simulink model "test_dram_vacc_147"  (R2012b)
settings: Solver=VariableStepDiscrete  SolverMode=SingleTasking  StartTime=0.0  StopTime=100000  RelTol=1e-3
undefined symbols (not defined in the file): blockCountBits, blockRowBits
libraries: xbsIndex_r4 x1042, xbsReplacements_r4 x87, casper_library_misc x9, xps_library x2
(part 2 of 9)

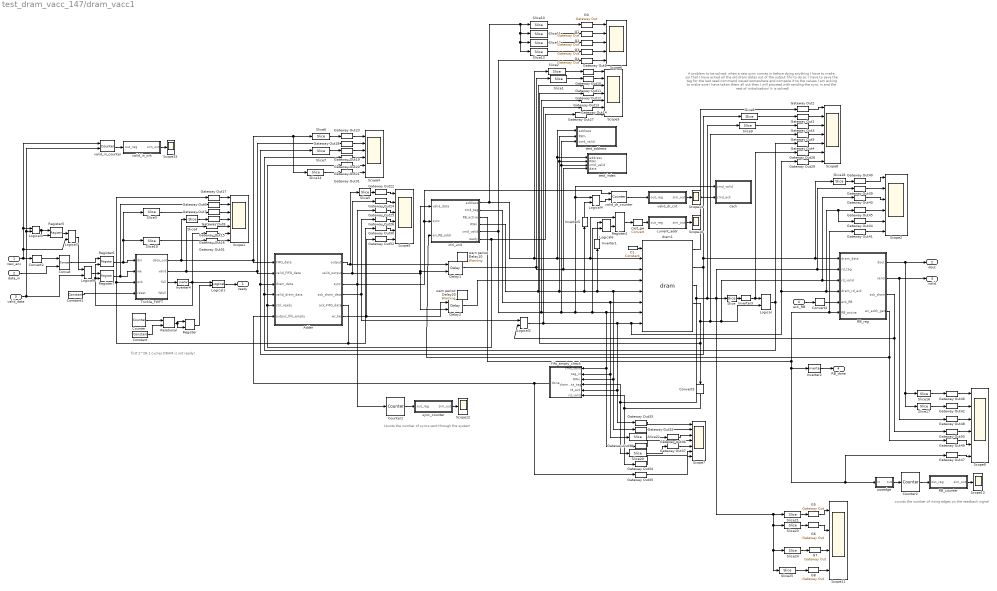
== system test_dram_vacc_147/dram_vacc1 ==
  note: counts the number of rising edges on
      | the readback signal
  note: counts the number of syncs
      | sent through the system
  note: first 2^28-1 cycles DRAM
      | is not ready!
  note: A problem to be solved:
      | when a new sync comes in before doing anything I have to make sur
      | that I have acked all the old dram datas out of the output fifo
      | to do so: I have to save the tag for the last read command issued somewhere
      | and compare it to the values I am acking to make sure I have taken them all out
      | then I will proceed with sending the sync in and the rest of initialization!
      | it is solved!
  new_acc : Inport
  data_in : Inport  Port=2
  valid_data : Inport  Port=3
  ack_RB : Inport  Port=4
  Adder : Subsystem
  C1 : xbsIndex_r4/Constant  const=0  gui_display_data_type=Fixed-point  arith_type=Boolean  n_bits=1  bin_pt=0  preci_type=Single  exp_width=8  frac_width=24  explicit_period=on  period=1  equ=P=C  opselect=C  inp2=PCIN>>17  opr=+  inp1=P  carry=CIN  dbl_ovrd=off  block_type=constant
  Concat : xbsIndex_r4/Concat  num_inputs=2  dbl_ovrd=off  block_type=concat
  Constant : xbsIndex_r4/Constant  const=2^28-1  gui_display_data_type=Fixed-point  arith_type=Unsigned  n_bits=28  bin_pt=0  preci_type=Single  exp_width=8  frac_width=24  explicit_period=on  period=1  equ=P=C  opselect=C  inp2=PCIN>>17  opr=+  inp1=P  carry=CIN  dbl_ovrd=off  block_type=constant
  Constant1 : xbsIndex_r4/Constant  const=0  gui_display_data_type=Fixed-point  arith_type=Boolean  n_bits=28  bin_pt=0  preci_type=Single  exp_width=8  frac_width=24  explicit_period=on  period=1  equ=P=C  opselect=C  inp2=PCIN>>17  opr=+  inp1=P  carry=CIN  dbl_ovrd=off  block_type=constant
  Convert2 : xbsIndex_r4/Convert  gui_display_data_type=Fixed-point  arith_type=Unsigned  n_bits=1  bin_pt=0  float_type=Single  exp_bits=8  fraction_bits=24  quantization=Truncate  overflow=Wrap  en=off  latency=0  dbl_ovrd=off  pipeline=off  block_type=convert
      settings: xl_area=[0, 0, 0, 0, 0, 0, 0]
  Convert3 : xbsIndex_r4/Convert  gui_display_data_type=Fixed-point  arith_type=Boolean  n_bits=31  bin_pt=0  float_type=Single  exp_bits=8  fraction_bits=24  quantization=Truncate  overflow=Wrap  en=off  latency=0  dbl_ovrd=off  pipeline=off  block_type=convert
      settings: xl_area=[0, 0, 0, 0, 0, 0, 0]
  Convert4 : xbsIndex_r4/Convert  gui_display_data_type=Fixed-point  arith_type=Boolean  n_bits=31  bin_pt=0  float_type=Single  exp_bits=8  fraction_bits=24  quantization=Truncate  overflow=Wrap  en=off  latency=0  dbl_ovrd=off  pipeline=off  block_type=convert
      settings: xl_area=[0, 0, 0, 0, 0, 0, 0]
  Counter : xbsIndex_r4/Counter  cnt_type=Free Running  cnt_to=Inf  operation=Up  start_count=0  cnt_by_val=1  arith_type=Unsigned  n_bits=28  bin_pt=0  load_pin=off  rst=off  en=off  explicit_period=off  period=1  dbl_ovrd=off  use_behavioral_HDL=off  implementation=Fabric  use_rpm=on  block_type=counter
      settings: xl_area=[0, 0, 0, 0, 0, 0, 0]
  Counter1 : xbsIndex_r4/Counter  cnt_type=Free Running  cnt_to=Inf  operation=Up  start_count=0  cnt_by_val=1  arith_type=Unsigned  n_bits=32  bin_pt=0  load_pin=off  rst=off  en=on  explicit_period=off  period=1  dbl_ovrd=off  use_behavioral_HDL=off  implementation=Fabric  use_rpm=on  block_type=counter
      settings: xl_area=[0, 0, 0, 0, 0, 0, 0]
  Counter2 : xbsIndex_r4/Counter  cnt_type=Free Running  cnt_to=Inf  operation=Up  start_count=0  cnt_by_val=1  arith_type=Unsigned  n_bits=32  bin_pt=0  load_pin=off  rst=off  en=on  explicit_period=off  period=1  dbl_ovrd=off  use_behavioral_HDL=off  implementation=Fabric  use_rpm=on  block_type=counter
      settings: xl_area=[0, 0, 0, 0, 0, 0, 0]
  Delay1 : xbsIndex_r4/Delay  rst=off  infoeditControl=Selection of Reset will increase slice count due to use of real FFs and instead of SRLs  en=on  latency=1  dbl_ovrd=off  reg_retiming=off  block_type=delay
      settings: xl_area=[0, 0, 0, 0, 0, 0, 0]
  Delay2 : xbsIndex_r4/Delay  rst=off  infoeditControl=Selection of Reset will increase slice count due to use of real FFs and instead of SRLs  en=on  latency=1  dbl_ovrd=off  reg_retiming=off  block_type=delay
      settings: xl_area=[0, 0, 0, 0, 0, 0, 0]
  G{0..8} (9 alike) : xbsIndex_r4/Gateway Out  inherit_from_input=off  hdl_port=off  timing_constraint=None  locs_specified=off  LOCs={}  UseAsDAC=off  DACChannel='1'  block_type=gatewayout
      settings: xl_area=[0, 0, 0, 0, 0, 0, 0]
  Gateway Out{1..52} (52 alike) : xbsIndex_r4/Gateway Out  inherit_from_input=off  hdl_port=off  timing_constraint=None  locs_specified=off  LOCs={}  UseAsDAC=off  DACChannel='1'  block_type=gatewayout
      settings: xl_area=[0, 0, 0, 0, 0, 0, 0]
  Inverter{1..5} (5 alike) : xbsIndex_r4/Inverter  en=off  latency=0  dbl_ovrd=off  block_type=inv
      settings: xl_area=[0, 0, 0, 0, 0, 0, 0]
  Logical{,1,3..4,6,8} (6 alike) : xbsIndex_r4/Logical  logical_function=AND  inputs=2  en=off  latency=0  precision=Full  arith_type=Unsigned  n_bits=8  bin_pt=2  align_bp=on  dbl_ovrd=off  block_type=logical
      settings: xl_area=[0, 0, 0, 0, 0, 0, 0]
  Logical2 : xbsIndex_r4/Logical  logical_function=OR  inputs=2  en=off  latency=0  precision=Full  arith_type=Unsigned  n_bits=8  bin_pt=2  align_bp=on  dbl_ovrd=off  block_type=logical
      settings: xl_area=[0, 0, 0, 0, 0, 0, 0]
  Logical7 : xbsIndex_r4/Logical  logical_function=OR  inputs=2  en=off  latency=0  precision=Full  arith_type=Unsigned  n_bits=8  bin_pt=2  align_bp=on  dbl_ovrd=off  block_type=logical
      settings: xl_area=[0, 0, 0, 0, 0, 0, 0]
  RB_counter : Subsystem  Tag=xps:sw_reg  AncestorBlock=xps_library/software register  mask(swreg){io_dir=To Processor, io_delay=0, sample_period=1, names=reg, bitwidths=32, bin_pts=0, arith_types=0, sim_port=on, show_format=on}
      mask prompts: io_dir "I/O direction"; io_delay "I/O delay"; sample_period "Sample period"; names "Bitfield names [msb...lsb]"; bitwidths "Bitfield widths"; bin_pts "Bitfield binary pts"; arith_types "Bitfield types, ufix=0, fix=1, bool=2"; sim_port "Provide sim input/output?"; show_format "Print format string?"
      mask help: A 32-bit software-accessible register. Can be divided into bitfields of varying widths and types using the fields in the block mask.
      mask init:
      | try
      |     swreg_init(gcb)
      | catch ex
      |     disp(sprintf('%s: %s', gcb, ex.message))
      |     errordlg(ex.message)
      | end
      settings: AttributesFormatString=1output:uf32.0
      mask TypeOptions io_dir: To Processor | From Processor
      mask Callback io_dir:
      | mask_enables = get_param(gcb, 'MaskEnables');
      | mask_names = get_param(gcb, 'MaskNames');
      | if strcmp(get_param(gcb, 'io_dir'), 'To Processor'),
      |     mask_enables{ismember(mask_names, 'sample_period')} = 'off';
      | else
      |     mask_enables{ismember(mask_names, 'sample_period')} = 'on';
      | end
      | set_param(gcb, 'MaskEnables', mask_enables);
  RB_reg : Subsystem
  Register{,2,5..7} (5 alike) : xbsIndex_r4/Register  init=0  rst=off  en=on  dbl_ovrd=off  block_type=register
      settings: xl_area=[0, 0, 0, 0, 0, 0, 0]
  Relational : xbsIndex_r4/Relational  mode=a=b  en=off  latency=1  dbl_ovrd=off  block_type=relational
      settings: xl_area=[0, 0, 0, 0, 0, 0, 0]
  Scope{1,3,7..8} (4 alike) : Scope  NumInputPorts=7
      Scope1 settings: TimeRange=30000  YMin=0~0~0.95~0.95~0~0.95~-1  YMax=1~1~1.05~1.05~1~1.05~1  SaveName=ScopeData7
      Scope3 settings: YMin=0~0~0~0~0~0~0  YMax=150~2500~1~1~1~1~1  SaveName=ScopeData6
      Scope7 settings: YMin=0~0~0~0~0~0.95~0  YMax=1~1100~7500~1~1~1.05~1  SaveName=ScopeData17
      Scope8 settings: YMin=0~0~2.68438e+008~0~0~0~0  YMax=1~11000~2.68439e+008~1~1~1~1  SaveName=ScopeData19
  Scope{10,12..15} (5 alike) : Scope
      Scope10 settings: YMin=0  YMax=100  SaveName=ScopeData27
      Scope12 settings: YMin=0  YMax=100  SaveName=ScopeData32
      Scope13 settings: YMin=0  YMax=100  SaveName=ScopeData33
      Scope14 settings: YMin=0  YMax=100  SaveName=ScopeData21
      Scope15 settings: YMin=0  YMax=100  SaveName=ScopeData24
  Scope11 : Scope  NumInputPorts=4
      settings: YMin=0~0.95~-1~1.9  YMax=120~1.05~1~2.1  SaveName=ScopeData28
  Scope{2,4..5,9} (4 alike) : Scope  NumInputPorts=6
      Scope2 settings: YMin=2.5~5e+008~0~0~0~0.95  YMax=12.5~2.75e+009~1~1~1~1.05  SaveName=ScopeData22
      Scope4 settings: YMin=0.95~0.95~-1~-1~0.95~-1  YMax=1.05~1.05~1~1~1.05~1  SaveName=ScopeData8
      Scope5 settings: YMin=0~0~-1~0~0~-5  YMax=250~1~1~1~1~5  SaveName=ScopeData9
      Scope9 settings: YMin=1.9~1.9~-1~0~-1~0.95  YMax=2.1~2.1~1~1~1~1.05  SaveName=ScopeData23
  Scope6 : Scope  NumInputPorts=5
      settings: YMin=0~0~0~0~0  YMax=200~4000~1~1~1  SaveName=ScopeData14
  Slice : xbsIndex_r4/Slice  nbits=1  boolean_output=on  mode=Upper Bit Location + Width  bit1=0  base1=MSB of Input  bit0=0  base0=LSB of Input  dbl_ovrd=off  block_type=slice
  Slice{1,3..8,16..18} (10 alike) : xbsIndex_r4/Slice  nbits=32  boolean_output=off  mode=Lower Bit Location + Width  bit1=0  base1=MSB of Input  bit0=0  base0=LSB of Input  dbl_ovrd=off  block_type=slice
  Slice{2,10,20,22} (4 alike) : xbsIndex_r4/Slice  nbits=8  boolean_output=off  mode=Lower Bit Location + Width  bit1=0  base1=MSB of Input  bit0=5  base0=LSB of Input  dbl_ovrd=off  block_type=slice
  Slice11 : xbsIndex_r4/Slice  nbits=14  boolean_output=off  mode=Lower Bit Location + Width  bit1=0  base1=MSB of Input  bit0=14  base0=LSB of Input  dbl_ovrd=off  block_type=slice
  Slice12 : xbsIndex_r4/Slice  nbits=1  boolean_output=off  mode=Lower Bit Location + Width  bit1=0  base1=MSB of Input  bit0=13  base0=LSB of Input  dbl_ovrd=off  block_type=slice
  Slice13 : xbsIndex_r4/Slice  nbits=2  boolean_output=off  mode=Lower Bit Location + Width  bit1=0  base1=MSB of Input  bit0=28  base0=LSB of Input  dbl_ovrd=off  block_type=slice
  Slice14 : xbsIndex_r4/Slice  nbits=1  boolean_output=off  mode=Upper Bit Location + Width  bit1=0  base1=MSB of Input  bit0=0  base0=LSB of Input  dbl_ovrd=off  block_type=slice
  Slice19 : xbsIndex_r4/Slice  nbits=1  boolean_output=off  mode=Upper Bit Location + Width  bit1=0  base1=MSB of Input  bit0=0  base0=LSB of Input  dbl_ovrd=off  block_type=slice
  Slice21 : xbsIndex_r4/Slice  nbits=8  boolean_output=off  mode=Lower Bit Location + Width  bit1=0  base1=MSB of Input  bit0=6  base0=LSB of Input  dbl_ovrd=off  block_type=slice
  Slice23 : xbsIndex_r4/Slice  nbits=14  boolean_output=off  mode=Lower Bit Location + Width  bit1=0  base1=MSB of Input  bit0=15  base0=LSB of Input  dbl_ovrd=off  block_type=slice
  Slice24 : xbsIndex_r4/Slice  nbits=1  boolean_output=off  mode=Lower Bit Location + Width  bit1=0  base1=MSB of Input  bit0=14  base0=LSB of Input  dbl_ovrd=off  block_type=slice
  Slice25 : xbsIndex_r4/Slice  nbits=2  boolean_output=off  mode=Lower Bit Location + Width  bit1=0  base1=MSB of Input  bit0=29  base0=LSB of Input  dbl_ovrd=off  block_type=slice
  Slice9 : xbsIndex_r4/Slice  nbits=31  boolean_output=off  mode=Lower Bit Location + Width  bit1=0  base1=MSB of Input  bit0=0  base0=LSB of Input  dbl_ovrd=off  block_type=slice
  Trickle_FWFT : Subsystem  mask{depth=512}
      mask init:
      | cursys = gcb ; 
      | set_param([cursys, '/FIFO'], 'depth', depth);
      mask TypeOptions depth: 16 | 32 | 64 | 128 | 256 | 512 | 1K | 2K | 4K | 8K | 16K | 32K | 64K
  cack : Subsystem
  cast_gw : xbsIndex_r4/Convert  gui_display_data_type=Fixed-point  arith_type=Unsigned  n_bits=32  bin_pt=0  float_type=Single  exp_bits=8  fraction_bits=24  quantization=Truncate  overflow=Wrap  en=off  latency=0  dbl_ovrd=off  pipeline=off  block_type=convert
  ctrl_unit : Subsystem  mask{burst_length=valid_length, acc_length=acc_length}
      mask prompts: burst_length "Burst Length?"; acc_length "Accumulation length?"
  current_addr : Subsystem  Tag=xps:sw_reg  AncestorBlock=xps_library/software register  mask(swreg){io_dir=To Processor, io_delay=0, sample_period=1, names=reg, bitwidths=32, bin_pts=0, arith_types=0, sim_port=on, show_format=on}
      mask prompts: io_dir "I/O direction"; io_delay "I/O delay"; sample_period "Sample period"; names "Bitfield names [msb...lsb]"; bitwidths "Bitfield widths"; bin_pts "Bitfield binary pts"; arith_types "Bitfield types, ufix=0, fix=1, bool=2"; sim_port "Provide sim input/output?"; show_format "Print format string?"
      mask help: A 32-bit software-accessible register. Can be divided into bitfields of varying widths and types using the fields in the block mask.
      mask init:
      | try
      |     swreg_init(gcb)
      | catch ex
      |     disp(sprintf('%s: %s', gcb, ex.message))
      |     errordlg(ex.message)
      | end
      settings: AttributesFormatString=1output:uf32.0
      mask TypeOptions io_dir: To Processor | From Processor
      mask Callback io_dir:
      | mask_enables = get_param(gcb, 'MaskEnables');
      | mask_names = get_param(gcb, 'MaskNames');
      | if strcmp(get_param(gcb, 'io_dir'), 'To Processor'),
      |     mask_enables{ismember(mask_names, 'sample_period')} = 'off';
      | else
      |     mask_enables{ismember(mask_names, 'sample_period')} = 'on';
      | end
      | set_param(gcb, 'MaskEnables', mask_enables);
  dram1 : xps_library/dram  Tag=xps:dram  dimm=1  arith_type=Unsigned  bin_pt=0  ip_clock=200  sample_period=1  bram_fifos=on  disable_tag=on  ram_depth=18  bank_mgt=on  wide_data=off  half_burst=off  use_sniffer=on
  fifo_empty_check : Subsystem
  posedge : Subsystem
  sync_counter : Subsystem  Tag=xps:sw_reg  AncestorBlock=xps_library/software register  mask(swreg){io_dir=To Processor, io_delay=0, sample_period=1, names=reg, bitwidths=32, bin_pts=0, arith_types=0, sim_port=on, show_format=on}
      mask prompts: io_dir "I/O direction"; io_delay "I/O delay"; sample_period "Sample period"; names "Bitfield names [msb...lsb]"; bitwidths "Bitfield widths"; bin_pts "Bitfield binary pts"; arith_types "Bitfield types, ufix=0, fix=1, bool=2"; sim_port "Provide sim input/output?"; show_format "Print format string?"
      mask help: A 32-bit software-accessible register. Can be divided into bitfields of varying widths and types using the fields in the block mask.
      mask init:
      | try
      |     swreg_init(gcb)
      | catch ex
      |     disp(sprintf('%s: %s', gcb, ex.message))
      |     errordlg(ex.message)
      | end
      settings: AttributesFormatString=1output:uf32.0
      mask TypeOptions io_dir: To Processor | From Processor
      mask Callback io_dir:
      | mask_enables = get_param(gcb, 'MaskEnables');
      | mask_names = get_param(gcb, 'MaskNames');
      | if strcmp(get_param(gcb, 'io_dir'), 'To Processor'),
      |     mask_enables{ismember(mask_names, 'sample_period')} = 'off';
      | else
      |     mask_enables{ismember(mask_names, 'sample_period')} = 'on';
      | end
      | set_param(gcb, 'MaskEnables', mask_enables);
  test_address : Subsystem
  test_index : Subsystem
  valid_dr_cnt : Subsystem  Tag=xps:sw_reg  AncestorBlock=xps_library/software register  mask(swreg){io_dir=To Processor, io_delay=0, sample_period=1, names=reg, bitwidths=32, bin_pts=0, arith_types=0, sim_port=on, show_format=on}
      mask prompts: io_dir "I/O direction"; io_delay "I/O delay"; sample_period "Sample period"; names "Bitfield names [msb...lsb]"; bitwidths "Bitfield widths"; bin_pts "Bitfield binary pts"; arith_types "Bitfield types, ufix=0, fix=1, bool=2"; sim_port "Provide sim input/output?"; show_format "Print format string?"
      mask help: A 32-bit software-accessible register. Can be divided into bitfields of varying widths and types using the fields in the block mask.
      mask init:
      | try
      |     swreg_init(gcb)
      | catch ex
      |     disp(sprintf('%s: %s', gcb, ex.message))
      |     errordlg(ex.message)
      | end
      settings: AttributesFormatString=1output:uf32.0
      mask TypeOptions io_dir: To Processor | From Processor
      mask Callback io_dir:
      | mask_enables = get_param(gcb, 'MaskEnables');
      | mask_names = get_param(gcb, 'MaskNames');
      | if strcmp(get_param(gcb, 'io_dir'), 'To Processor'),
      |     mask_enables{ismember(mask_names, 'sample_period')} = 'off';
      | else
      |     mask_enables{ismember(mask_names, 'sample_period')} = 'on';
      | end
      | set_param(gcb, 'MaskEnables', mask_enables);
  valid_dr_counter : xbsIndex_r4/Counter  cnt_type=Count Limited  cnt_to=Inf  operation=Up  start_count=0  cnt_by_val=1  arith_type=Unsigned  n_bits=32  bin_pt=0  load_pin=off  rst=on  en=on  explicit_period=off  period=1  dbl_ovrd=off  use_behavioral_HDL=off  implementation=Fabric  use_rpm=on  block_type=counter
      settings: xl_area=[0, 0, 0, 0, 0, 0, 0]
  valid_in_cnt : Subsystem  Tag=xps:sw_reg  AncestorBlock=xps_library/software register  mask(swreg){io_dir=To Processor, io_delay=0, sample_period=1, names=reg, bitwidths=32, bin_pts=0, arith_types=0, sim_port=on, show_format=on}
      mask prompts: io_dir "I/O direction"; io_delay "I/O delay"; sample_period "Sample period"; names "Bitfield names [msb...lsb]"; bitwidths "Bitfield widths"; bin_pts "Bitfield binary pts"; arith_types "Bitfield types, ufix=0, fix=1, bool=2"; sim_port "Provide sim input/output?"; show_format "Print format string?"
      mask help: A 32-bit software-accessible register. Can be divided into bitfields of varying widths and types using the fields in the block mask.
      mask init:
      | try
      |     swreg_init(gcb)
      | catch ex
      |     disp(sprintf('%s: %s', gcb, ex.message))
      |     errordlg(ex.message)
      | end
      settings: AttributesFormatString=1output:uf32.0
      mask TypeOptions io_dir: To Processor | From Processor
      mask Callback io_dir:
      | mask_enables = get_param(gcb, 'MaskEnables');
      | mask_names = get_param(gcb, 'MaskNames');
      | if strcmp(get_param(gcb, 'io_dir'), 'To Processor'),
      |     mask_enables{ismember(mask_names, 'sample_period')} = 'off';
      | else
      |     mask_enables{ismember(mask_names, 'sample_period')} = 'on';
      | end
      | set_param(gcb, 'MaskEnables', mask_enables);
  valid_in_counter : xbsIndex_r4/Counter  cnt_type=Count Limited  cnt_to=Inf  operation=Up  start_count=0  cnt_by_val=1  arith_type=Unsigned  n_bits=32  bin_pt=0  load_pin=off  rst=on  en=on  explicit_period=off  period=1  dbl_ovrd=off  use_behavioral_HDL=off  implementation=Fabric  use_rpm=on  block_type=counter
      settings: xl_area=[0, 0, 0, 0, 0, 0, 0]
  warn period Delay10 : xbsReplacements_r4/Warning  period=1
  warn period Delay20 : xbsReplacements_r4/Warning  period=1
  ready : Outport
  dout : Outport  Port=2
  valid : Outport  Port=3
  RB_done : Outport  Port=4
  wires:
  Convert4/1 -> RB_reg/5(ack_RB)
  Inverter3/1 -> Gateway Out28/1, Logical/1
  ack_RB/1 -> Convert4/1
  ctrl_unit/5(cmd_valid) -> G4/1, Gateway Out13/1, dram1/7, Gateway Out38/1, fifo_empty_check/1(cmd_valid), Logical6/2, cack/1(cmd_valid), Logical4/1, test_address/3(cmd_valid), test_index/3(cmd_valid)
  Inverter2/1 -> RB_done/1
  posedge/1(out) -> Counter2/1
  RB_counter/1(sim_out) -> Scope13/1
  Counter2/1 -> RB_counter/1(out_reg)
  sync_counter/1(sim_out) -> Scope12/1
  Counter1/1 -> sync_counter/1(out_reg)
  Inverter4/1 -> Logical1/1, Gateway Out16/1, Register7/2, Register6/2
  G8/1 -> Scope11/4
  G7/1 -> Scope11/3
  G6/1 -> Scope11/2
  G5/1 -> Scope11/1
  Slice25/1 -> G8/1
  Slice24/1 -> G7/1
  Slice23/1 -> G6/1
  Slice21/1 -> G5/1
  Slice20/1 -> Gateway Out37/1
  Slice22/1 -> Gateway Out36/1
  current_addr/1(sim_out) -> Scope10/1
  Inverter1/1 -> Logical6/1
  Logical6/1 -> Register2/2
  Register2/1 -> cast_gw/1
  Slice19/1 -> Gateway Out51/1
  Gateway Out51/1 -> Scope1/7
  Register7/1 -> Gateway Out6/1, Trickle_FWFT/2(we)
  Register/1 -> Logical1/2
  Relational/1 -> Register/2, Register/1
  Constant/1 -> Relational/2
  Counter/1 -> Relational/1
  Logical1/1 -> ready/1
  Gateway Out47/1 -> Scope9/6
  Slice18/1 -> Gateway Out40/1
  Slice17/1 -> Gateway Out42/1
  Slice16/1 -> Gateway Out46/1
  Convert3/1 -> Gateway Out34/1, fifo_empty_check/6(rd_valid)
  Gateway Out49/1 -> Scope9/5
  Gateway Out50/1 -> Scope9/4
  Gateway Out48/1 -> Scope9/3
  Gateway Out42/1 -> Scope9/2
  Gateway Out46/1 -> Scope9/1
  Gateway Out41/1 -> Scope2/6
  Gateway Out44/1 -> Scope2/5
  Gateway Out45/1 -> Scope2/4
  Gateway Out43/1 -> Scope2/3
  Gateway Out39/1 -> Scope2/2
  Gateway Out40/1 -> Scope2/1
  Logical2/1 -> Gateway Out14/1, dram1/8, Gateway Out44/1, Gateway Out45/1, RB_reg/4(dram_rd_ack), Gateway Out29/1, Gateway Out33/1, fifo_empty_check/5(rd_ack)
  ctrl_unit/3(RB_active) -> Inverter2/1, posedge/1(in), Gateway Out47/1, RB_reg/6(RB_active), Gateway Out41/1
  RB_reg/4(en_addr_gen) -> Gateway Out49/1, ctrl_unit/3(en_RB_addr)
  RB_reg/3(ack_dram) -> Logical2/2, Gateway Out50/1
  RB_reg/2(valid) -> valid/1, Gateway Out48/1
  RB_reg/1(dout) -> Slice17/1, Slice16/1, dout/1
  Gateway Out29/1 -> Scope8/7
  Gateway Out28/1 -> Scope8/6
  Gateway Out4/1 -> Scope8/5
  Gateway Out5/1 -> Scope8/4
  Gateway Out3/1 -> Scope8/3
  Gateway Out1/1 -> Scope8/2
  Gateway Out2/1 -> Scope8/1
  Gateway Out35/1 -> Scope7/7
  Gateway Out34/1 -> Scope7/6
  Gateway Out38/1 -> Scope7/4
  Gateway Out37/1 -> Scope7/5
  Gateway Out36/1 -> Scope7/3
  Gateway Out32/1 -> Scope7/2
  Gateway Out33/1 -> Scope7/1
  fifo_empty_check/1(done) -> Gateway Out35/1, Adder/6(output_fifo_empty)
  Delay1/1 -> Slice1/1, dram1/3, test_index/4(data)
  Slice14/1 -> Gateway Out31/1
  Gateway Out31/1 -> Scope4/6
  G4/1 -> Scope6/5
  G3/1 -> Scope6/4
  G2/1 -> Scope6/3
  G1/1 -> Scope6/2
  G0/1 -> Scope6/1
  Slice13/1 -> G3/1
  Slice12/1 -> G2/1
  Slice11/1 -> G1/1
  Slice10/1 -> G0/1
  Gateway Out30/1 -> Scope5/5
  Adder/5(ack_FIFO_data) -> Gateway Out30/1, Gateway Out17/1, Trickle_FWFT/3(ack)
  Slice9/1 -> Gateway Out3/1
  Slice8/1 -> Gateway Out1/1
  Gateway Out27/1 -> Scope3/7
  Slice7/1 -> Gateway Out19/1
  Slice6/1 -> Gateway Out23/1
  Slice5/1 -> Gateway Out22/1
  Logical/1 -> Adder/4(valid_dram_data), Gateway Out20/1, Gateway Out4/1
  Slice4/1 -> Gateway Out8/1
  Slice3/1 -> Gateway Out7/1
  Gateway Out26/1 -> Scope5/4
  Gateway Out25/1 -> Scope5/3
  Gateway Out24/1 -> Scope5/2
  Gateway Out22/1 -> Scope5/1
  Gateway Out21/1 -> Scope4/5
  Gateway Out20/1 -> Scope4/4
  Gateway Out19/1 -> Scope4/3
  Gateway Out18/1 -> Scope4/2
  Gateway Out23/1 -> Scope4/1
  Gateway Out16/1 -> Scope1/6
  Gateway Out15/1 -> Scope1/5
  Gateway Out8/1 -> Scope1/4
  Gateway Out7/1 -> Scope1/3
  Gateway Out6/1 -> Scope1/2
  Gateway Out17/1 -> Scope1/1
  Slice2/1 -> Gateway Out9/1
  Slice1/1 -> Gateway Out10/1
  Gateway Out14/1 -> Scope3/6
  Gateway Out13/1 -> Scope3/5
  Gateway Out12/1 -> Scope3/4
  Gateway Out11/1 -> Scope3/3
  Gateway Out10/1 -> Scope3/2
  Gateway Out9/1 -> Scope3/1
  Register6/1 -> Slice19/1, Slice3/1, Trickle_FWFT/1(din)
  Trickle_FWFT/3(full) -> Inverter4/1
  ctrl_unit/2(cmd_tag) -> dram1/6, Slice22/1, fifo_empty_check/2(tag_in)
  dram1/1 -> Gateway Out2/1, cack/2(cmd_ack)
  Adder/3(sync) -> Counter1/1, ctrl_unit/2(sync), valid_dr_counter/1, Gateway Out25/1
  Adder/2(valid_output) -> Gateway Out24/1, Delay1/2, ctrl_unit/1(valid_data), Delay2/2
  ctrl_unit/6(ready) -> Gateway Out27/1, Adder/5(ctrl_ready), Gateway Out21/1
  dram1/4 -> Convert3/1, Gateway Out12/1, RB_reg/3(rd_valid), Gateway Out43/1, Logical/2, Gateway Out5/1
  Slice/1 -> Inverter3/1
  dram1/3 -> Slice20/1, fifo_empty_check/4(dram_data_tag), RB_reg/2(rd_tag), Gateway Out39/1, Slice/1, Slice24/1, Slice25/1, Slice23/1, Slice21/1, Slice9/1
  dram1/2 -> Adder/3(dram_data), Slice7/1, RB_reg/1(dram_data), Slice18/1, Slice8/1
  Adder/1(output) -> Delay1/1, Slice5/1
  C1/1 -> dram1/1
  ctrl_unit/4(RWn) -> Gateway Out11/1, Inverter1/1, dram1/5, Gateway Out32/1, fifo_empty_check/3(RWn), Inverter5/1, test_address/2(RWn), test_index/2(RWn)
  ctrl_unit/1(address) -> Slice2/1, dram1/2, Register2/1, test_address/1(address), test_index/1(address), Slice12/1, Slice13/1, Slice11/1, Slice10/1
  Trickle_FWFT/2(valid) -> Adder/2(valid_FIFO_data), Gateway Out18/1, Gateway Out15/1
  Trickle_FWFT/1(data_out) -> Slice4/1, Slice14/1, Slice6/1, Adder/1(FIFO_data)
  Adder/4(ack_dram_data) -> Logical2/1, Gateway Out26/1
  new_acc/1 -> Convert2/1, Logical7/2, Logical3/1, valid_in_counter/1
  data_in/1 -> Concat/2
  valid_data/1 -> Logical8/2, Logical3/2, valid_in_counter/2
  Convert2/1 -> Concat/1
  Register5/1 -> Logical7/1
  Logical7/1 -> Logical8/1
  Logical3/1 -> Register5/1, Register5/2
  Concat/1 -> Register6/1
  Logical8/1 -> Register7/1
  Constant1/1 -> Trickle_FWFT/4(reset)
  Logical4/1 -> valid_dr_counter/2
  valid_dr_cnt/1(sim_out) -> Scope14/1
  valid_dr_counter/1 -> valid_dr_cnt/1(out_reg)
  Inverter5/1 -> Logical4/2
  valid_in_cnt/1(sim_out) -> Scope15/1
  valid_in_counter/1 -> valid_in_cnt/1(out_reg)
  Adder/6(wr_be) -> Delay2/1, Gateway Out52/1
  Delay2/1 -> dram1/4
  Gateway Out52/1 -> Scope5/6
  cast_gw/1 -> current_addr/1(out_reg)

== system test_dram_vacc_147/rb_done ==
  out_reg : Inport
  assert_reg : xbsIndex_r4/Assert  assert_type=on  type_source=Explicitly  gui_display_data_type=Boolean  arith_type=Boolean  n_bits=1  bin_pt=0  preci_type=Single  exp_width=8  frac_width=24  assert_rate=off  rate_source=Explicitly  period=1  output_port=on  block_type=assert
  cast_gw : xbsIndex_r4/Convert  gui_display_data_type=Fixed-point  arith_type=Unsigned  n_bits=32  bin_pt=0  float_type=Single  exp_bits=8  fraction_bits=24  quantization=Truncate  overflow=Wrap  en=off  latency=0  dbl_ovrd=off  pipeline=off  block_type=convert
  io_delay : xbsIndex_r4/Delay  rst=off  infoeditControl=Selection of Reset will increase slice count due to use of real FFs and instead of SRLs  en=off  latency=0  dbl_ovrd=off  reg_retiming=on  block_type=delay
  reint1 : xbsIndex_r4/Reinterpret  force_arith_type=on  arith_type=Unsigned  force_bin_pt=on  bin_pt=0  block_type=reinterpret
  test_dram_vacc_147_rb_done_user_data_in : xbsIndex_r4/Gateway Out  inherit_from_input=off  hdl_port=on  timing_constraint=None  locs_specified=off  LOCs={}  UseAsDAC=off  DACChannel='1'  block_type=gatewayout
  sim_out : Outport
  wires:
  io_delay/1 -> cast_gw/1
  cast_gw/1 -> test_dram_vacc_147_rb_done_user_data_in/1
  test_dram_vacc_147_rb_done_user_data_in/1 -> sim_out/1
  out_reg/1 -> assert_reg/1
  assert_reg/1 -> reint1/1
  reint1/1 -> io_delay/1

== system test_dram_vacc_147/ready ==
  out_reg : Inport
  assert_reg : xbsIndex_r4/Assert  assert_type=on  type_source=Explicitly  gui_display_data_type=Boolean  arith_type=Boolean  n_bits=1  bin_pt=0  preci_type=Single  exp_width=8  frac_width=24  assert_rate=off  rate_source=Explicitly  period=1  output_port=on  block_type=assert
  cast_gw : xbsIndex_r4/Convert  gui_display_data_type=Fixed-point  arith_type=Unsigned  n_bits=32  bin_pt=0  float_type=Single  exp_bits=8  fraction_bits=24  quantization=Truncate  overflow=Wrap  en=off  latency=0  dbl_ovrd=off  pipeline=off  block_type=convert
  io_delay : xbsIndex_r4/Delay  rst=off  infoeditControl=Selection of Reset will increase slice count due to use of real FFs and instead of SRLs  en=off  latency=0  dbl_ovrd=off  reg_retiming=on  block_type=delay
  reint1 : xbsIndex_r4/Reinterpret  force_arith_type=on  arith_type=Unsigned  force_bin_pt=on  bin_pt=0  block_type=reinterpret
  test_dram_vacc_147_ready_user_data_in : xbsIndex_r4/Gateway Out  inherit_from_input=off  hdl_port=on  timing_constraint=None  locs_specified=off  LOCs={}  UseAsDAC=off  DACChannel='1'  block_type=gatewayout
  sim_out : Outport
  wires:
  io_delay/1 -> cast_gw/1
  cast_gw/1 -> test_dram_vacc_147_ready_user_data_in/1
  test_dram_vacc_147_ready_user_data_in/1 -> sim_out/1
  out_reg/1 -> assert_reg/1
  assert_reg/1 -> reint1/1
  reint1/1 -> io_delay/1

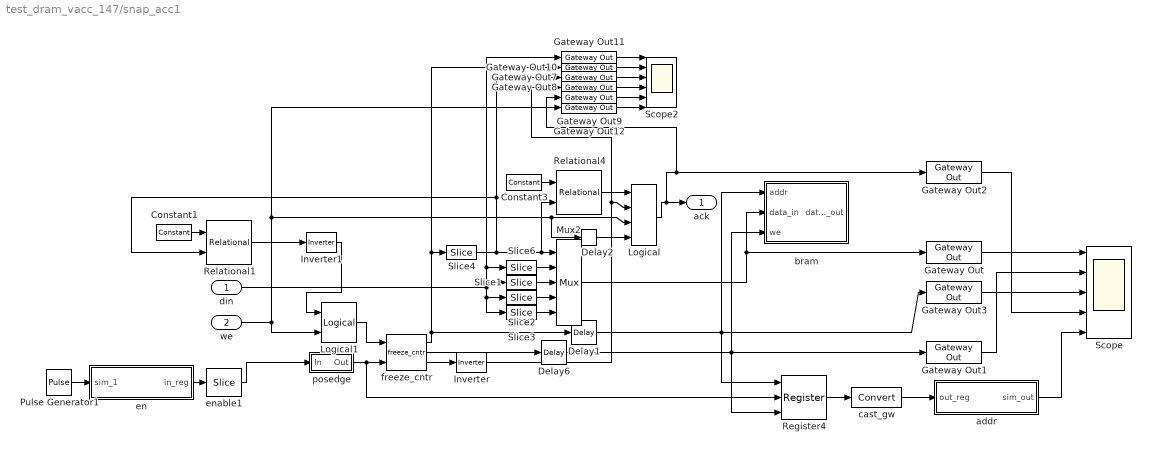
== system test_dram_vacc_147/snap_acc1 ==
  din : Inport
  we : Inport  Port=2
  Constant1 : xbsIndex_r4/Constant  const=0  gui_display_data_type=Fixed-point  arith_type=Unsigned  n_bits=2  bin_pt=0  preci_type=Single  exp_width=8  frac_width=24  explicit_period=on  period=1  equ=P=C  opselect=C  inp2=PCIN>>17  opr=+  inp1=P  carry=CIN  dbl_ovrd=off  block_type=constant
  Constant3 : xbsIndex_r4/Constant  const=3  gui_display_data_type=Fixed-point  arith_type=Unsigned  n_bits=2  bin_pt=0  preci_type=Single  exp_width=8  frac_width=24  explicit_period=on  period=1  equ=P=C  opselect=C  inp2=PCIN>>17  opr=+  inp1=P  carry=CIN  dbl_ovrd=off  block_type=constant
  Delay1 : xbsIndex_r4/Delay  rst=off  infoeditControl=Selection of Reset will increase slice count due to use of real FFs and instead of SRLs  en=off  latency=2  dbl_ovrd=off  reg_retiming=off  block_type=delay
      settings: xl_area=[0, 0, 0, 0, 0, 0, 0]
  Delay2 : xbsIndex_r4/Delay  rst=off  infoeditControl=Selection of Reset will increase slice count due to use of real FFs and instead of SRLs  en=off  latency=1  dbl_ovrd=off  reg_retiming=off  block_type=delay
      settings: xl_area=[0, 0, 0, 0, 0, 0, 0]
  Delay6 : xbsIndex_r4/Delay  rst=off  infoeditControl=Selection of Reset will increase slice count due to use of real FFs and instead of SRLs  en=off  latency=2  dbl_ovrd=off  reg_retiming=off  block_type=delay
      settings: xl_area=[0, 0, 0, 0, 0, 0, 0]
  Gateway Out{,1..3,7..12} (10 alike) : xbsIndex_r4/Gateway Out  inherit_from_input=off  hdl_port=off  timing_constraint=None  locs_specified=off  LOCs={}  UseAsDAC=off  DACChannel='1'  block_type=gatewayout
      settings: xl_area=[0, 0, 0, 0, 0, 0, 0]
  Inverter : xbsIndex_r4/Inverter  en=off  latency=0  dbl_ovrd=off  block_type=inv
      settings: xl_area=[0, 0, 0, 0, 0, 0, 0]
  Inverter1 : xbsIndex_r4/Inverter  en=off  latency=0  dbl_ovrd=off  block_type=inv
      settings: xl_area=[0, 0, 0, 0, 0, 0, 0]
  Logical : xbsIndex_r4/Logical  logical_function=AND  inputs=4  en=off  latency=0  precision=Full  arith_type=Unsigned  n_bits=8  bin_pt=2  align_bp=on  dbl_ovrd=off  block_type=logical
      settings: xl_area=[0, 0, 0, 0, 0, 0, 0]
  Logical1 : xbsIndex_r4/Logical  logical_function=OR  inputs=2  en=off  latency=0  precision=Full  arith_type=Unsigned  n_bits=8  bin_pt=2  align_bp=on  dbl_ovrd=off  block_type=logical
      settings: xl_area=[0, 0, 0, 0, 0, 0, 0]
  Mux2 : xbsIndex_r4/Mux  inputs=4  en=off  latency=2  precision=Full  arith_type="Signed  (2's comp)"  n_bits=8  bin_pt=2  quantization=Truncate  overflow=Wrap  dbl_ovrd=off  block_type=mux
      settings: xl_area=[0, 0, 0, 0, 0, 0, 0]
  Pulse Generator1 : DiscretePulseGenerator  Period=100  PulseWidth=5
  Register4 : xbsIndex_r4/Register  init=0  rst=on  en=on  dbl_ovrd=off  block_type=register
      settings: xl_area=[0, 0, 0, 0, 0, 0, 0]
  Relational1 : xbsIndex_r4/Relational  mode=a=b  en=off  latency=0  dbl_ovrd=off  block_type=relational
      settings: xl_area=[0, 0, 0, 0, 0, 0, 0]
  Relational4 : xbsIndex_r4/Relational  mode=a=b  en=off  latency=0  dbl_ovrd=off  block_type=relational
      settings: xl_area=[0, 0, 0, 0, 0, 0, 0]
  Scope : Scope  NumInputPorts=5
      settings: YMin=0~0~0~0~0  YMax=3.5e+009~1~175~1~175
  Scope2 : Scope  NumInputPorts=6
      settings: YMin=0~0~0~-5~-5~-5  YMax=3.5e+009~1~175~5~5~5  SaveName=ScopeData2
  Slice1 : xbsIndex_r4/Slice  nbits=32  boolean_output=off  mode=Upper Bit Location + Width  bit1=-32  base1=MSB of Input  bit0=0  base0=LSB of Input  dbl_ovrd=off  block_type=slice
  Slice2 : xbsIndex_r4/Slice  nbits=32  boolean_output=off  mode=Upper Bit Location + Width  bit1=-64  base1=MSB of Input  bit0=0  base0=LSB of Input  dbl_ovrd=off  block_type=slice
  Slice3 : xbsIndex_r4/Slice  nbits=32  boolean_output=off  mode=Upper Bit Location + Width  bit1=-96  base1=MSB of Input  bit0=0  base0=LSB of Input  dbl_ovrd=off  block_type=slice
  Slice4 : xbsIndex_r4/Slice  nbits=2  boolean_output=off  mode=Lower Bit Location + Width  bit1=0  base1=MSB of Input  bit0=0  base0=LSB of Input  dbl_ovrd=off  block_type=slice
  Slice6 : xbsIndex_r4/Slice  nbits=32  boolean_output=off  mode=Upper Bit Location + Width  bit1=0  base1=MSB of Input  bit0=0  base0=LSB of Input  dbl_ovrd=off  block_type=slice
  addr : Subsystem  Tag=xps:sw_reg  AncestorBlock=xps_library/software register  mask(swreg){io_dir=To Processor, io_delay=0, sample_period=1, names=reg, bitwidths=32, bin_pts=0, arith_types=0, sim_port=on, show_format=on}
      mask prompts: io_dir "I/O direction"; io_delay "I/O delay"; sample_period "Sample period"; names "Bitfield names [msb...lsb]"; bitwidths "Bitfield widths"; bin_pts "Bitfield binary pts"; arith_types "Bitfield types, ufix=0, fix=1, bool=2"; sim_port "Provide sim input/output?"; show_format "Print format string?"
      mask help: A 32-bit software-accessible register. Can be divided into bitfields of varying widths and types using the fields in the block mask.
      mask init:
      | try
      |     swreg_init(gcb)
      | catch ex
      |     disp(sprintf('%s: %s', gcb, ex.message))
      |     errordlg(ex.message)
      | end
      settings: AttributesFormatString=1output:uf32.0
      mask TypeOptions io_dir: To Processor | From Processor
      mask Callback io_dir:
      | mask_enables = get_param(gcb, 'MaskEnables');
      | mask_names = get_param(gcb, 'MaskNames');
      | if strcmp(get_param(gcb, 'io_dir'), 'To Processor'),
      |     mask_enables{ismember(mask_names, 'sample_period')} = 'off';
      | else
      |     mask_enables{ismember(mask_names, 'sample_period')} = 'on';
      | end
      | set_param(gcb, 'MaskEnables', mask_enables);
  bram : Subsystem  Tag=xps:bram  AncestorBlock=xps_library/Shared BRAM  mask{arith_type=Unsigned, addr_width=11, data_width=32, reg_prim_output=off, reg_core_output=off, optimization=Minimum_Area, data_bin_pt=0, init_vals=0, sample_rate=1}
      mask prompts: arith_type "Output Data Type"; addr_width "Address width"; data_width "Data Width"; reg_prim_output "Register Primitive Output"; reg_core_output "Register Core Output"; data_bin_pt "Data Binary Point"; init_vals "Initial values (simulation only)"; sample_rate "Sample rate"
      mask init:
      | shared_bram_mask;
      mask TypeOptions arith_type: Unsigned | Signed  (2's comp)
      mask TypeOptions data_width: 8 | 16 | 32 | 64 | 128
      mask TypeOptions optimization: Minimum_Area | Low_Power
  cast_gw : xbsIndex_r4/Convert  gui_display_data_type=Fixed-point  arith_type=Unsigned  n_bits=32  bin_pt=0  float_type=Single  exp_bits=8  fraction_bits=24  quantization=Truncate  overflow=Wrap  en=off  latency=0  dbl_ovrd=off  pipeline=off  block_type=convert
  en : Subsystem  Tag=xps:sw_reg  AncestorBlock=xps_library/software register  mask(swreg){io_dir=From Processor, io_delay=0, sample_period=1, names=reg, bitwidths=32, bin_pts=0, arith_types=0, sim_port=on, show_format=on}
      mask prompts: io_dir "I/O direction"; io_delay "I/O delay"; sample_period "Sample period"; names "Bitfield names [msb...lsb]"; bitwidths "Bitfield widths"; bin_pts "Bitfield binary pts"; arith_types "Bitfield types, ufix=0, fix=1, bool=2"; sim_port "Provide sim input/output?"; show_format "Print format string?"
      mask help: A 32-bit software-accessible register. Can be divided into bitfields of varying widths and types using the fields in the block mask.
      mask init:
      | try
      |     swreg_init(gcb)
      | catch ex
      |     disp(sprintf('%s: %s', gcb, ex.message))
      |     errordlg(ex.message)
      | end
      settings: AttributesFormatString=1input:uf32.0
      mask TypeOptions io_dir: To Processor | From Processor
      mask Callback io_dir:
      | mask_enables = get_param(gcb, 'MaskEnables');
      | mask_names = get_param(gcb, 'MaskNames');
      | if strcmp(get_param(gcb, 'io_dir'), 'To Processor'),
      |     mask_enables{ismember(mask_names, 'sample_period')} = 'off';
      | else
      |     mask_enables{ismember(mask_names, 'sample_period')} = 'on';
      | end
      | set_param(gcb, 'MaskEnables', mask_enables);
  enable1 : xbsIndex_r4/Slice  nbits=1  boolean_output=on  mode=Lower Bit Location + Width  bit1=0  base1=LSB of Input  bit0=0  base0=LSB of Input  dbl_ovrd=off  block_type=slice
  freeze_cntr : casper_library_misc/freeze_cntr  CounterBits=11
  posedge : Subsystem  Tag=Rising Edge Detector
  ack : Outport
  wires:
  Gateway Out1/1 -> Scope/2
  Gateway Out/1 -> Scope/1
  freeze_cntr/1 -> Slice4/1, Gateway Out10/1, Delay1/1
  enable1/1 -> posedge/1(In)
  posedge/1(Out) -> freeze_cntr/2, Register4/2
  freeze_cntr/2 -> Delay6/1
  Register4/1 -> cast_gw/1
  Mux2/1 -> bram/2(data_in), Gateway Out/1
  Slice6/1 -> Mux2/2
  Slice1/1 -> Mux2/3
  Slice2/1 -> Mux2/4
  Slice3/1 -> Mux2/5
  din/1 -> Slice1/1, Slice6/1, Gateway Out11/1, Slice2/1, Slice3/1
  Slice4/1 -> Relational4/2, Mux2/1, Gateway Out7/1, Relational1/2
  Constant3/1 -> Relational4/1
  Relational4/1 -> Logical/1
  Delay6/1 -> Register4/3, bram/3(we), Gateway Out1/1
  Delay1/1 -> Register4/1, bram/1(addr), Gateway Out3/1
  Gateway Out2/1 -> Scope/4
  Gateway Out3/1 -> Scope/3
  addr/1(sim_out) -> Scope/5
  Logical/1 -> Gateway Out2/1, Gateway Out9/1, ack/1
  freeze_cntr/3 -> Inverter/1
  Inverter/1 -> Logical/2, Gateway Out8/1
  Pulse Generator1/1 -> en/1(sim_1)
  en/1(in_reg) -> enable1/1
  we/1 -> Logical1/2, Gateway Out12/1, Logical/3, Delay2/1
  Gateway Out7/1 -> Scope2/3
  Gateway Out8/1 -> Scope2/4
  Gateway Out9/1 -> Scope2/5
  Gateway Out10/1 -> Scope2/2
  Gateway Out11/1 -> Scope2/1
  Gateway Out12/1 -> Scope2/6
  Logical1/1 -> freeze_cntr/1
  Inverter1/1 -> Logical1/1
  Delay2/1 -> Logical/4
  Constant1/1 -> Relational1/1
  Relational1/1 -> Inverter1/1
  cast_gw/1 -> addr/1(out_reg)

== system test_dram_vacc_147/tvg_sel ==
  sim_1 : Inport
  io_delay : xbsIndex_r4/Delay  rst=off  infoeditControl=Selection of Reset will increase slice count due to use of real FFs and instead of SRLs  en=off  latency=0  dbl_ovrd=off  reg_retiming=on  block_type=delay
  reint1 : xbsIndex_r4/Reinterpret  force_arith_type=on  arith_type=Unsigned  force_bin_pt=on  bin_pt=0  block_type=reinterpret
  slice_reg : xbsIndex_r4/Slice  nbits=32  boolean_output=off  mode=Lower Bit Location + Width  bit1=0  base1=MSB of Input  bit0=0  base0=LSB of Input  dbl_ovrd=off  block_type=slice
  test_dram_vacc_147_tvg_sel_user_data_out : xbsIndex_r4/Gateway In  gui_display_data_type=Fixed-point  arith_type=Unsigned  n_bits=32  bin_pt=0  preci_type=Single  exp_width=8  frac_width=24  quantization="Round  (unbiased: +/- Inf)"  overflow=Saturate  period=1  dbl_ovrd=off  timing_constraint=None  locs_specified=off  LOCs={}  UseAsADC=off  ADCChannel='1'  inherit_from_input=off  hdl_port=on  block_type=gatewayin
  in_reg : Outport
  wires:
  test_dram_vacc_147_tvg_sel_user_data_out/1 -> io_delay/1
  sim_1/1 -> test_dram_vacc_147_tvg_sel_user_data_out/1
  io_delay/1 -> slice_reg/1
  slice_reg/1 -> reint1/1
  reint1/1 -> in_reg/1

== system test_dram_vacc_147/Subsystem/data_sel1 ==
  In1 : Inport
  Product : Product  RndMeth=Zero
  err_clear_sim1 : Constant  Value=2^bit_pos
  Out1 : Outport
  wires:
  err_clear_sim1/1 -> Product/2
  In1/1 -> Product/1
  Product/1 -> Out1/1

== system test_dram_vacc_147/Subsystem/inj_counter1 ==
  In1 : Inport
  Product : Product  RndMeth=Zero
  err_clear_sim1 : Constant  Value=2^bit_pos
  Out1 : Outport
  wires:
  err_clear_sim1/1 -> Product/2
  In1/1 -> Product/1
  Product/1 -> Out1/1

== system test_dram_vacc_147/Subsystem/inj_vector1 ==
  In1 : Inport
  Product : Product  RndMeth=Zero
  err_clear_sim1 : Constant  Value=2^bit_pos
  Out1 : Outport
  wires:
  err_clear_sim1/1 -> Product/2
  In1/1 -> Product/1
  Product/1 -> Out1/1

== system test_dram_vacc_147/Subsystem/new_acc2 ==
  In1 : Inport
  Product : Product  RndMeth=Zero
  err_clear_sim1 : Constant  Value=2^bit_pos
  Out1 : Outport
  wires:
  err_clear_sim1/1 -> Product/2
  In1/1 -> Product/1
  Product/1 -> Out1/1

== system test_dram_vacc_147/Subsystem/run1 ==
  In1 : Inport
  Product : Product  RndMeth=Zero
  err_clear_sim1 : Constant  Value=2^bit_pos
  Out1 : Outport
  wires:
  err_clear_sim1/1 -> Product/2
  In1/1 -> Product/1
  Product/1 -> Out1/1

== system test_dram_vacc_147/Subsystem/valid_sel1 ==
  In1 : Inport
  Product : Product  RndMeth=Zero
  err_clear_sim1 : Constant  Value=2^bit_pos
  Out1 : Outport
  wires:
  err_clear_sim1/1 -> Product/2
  In1/1 -> Product/1
  Product/1 -> Out1/1

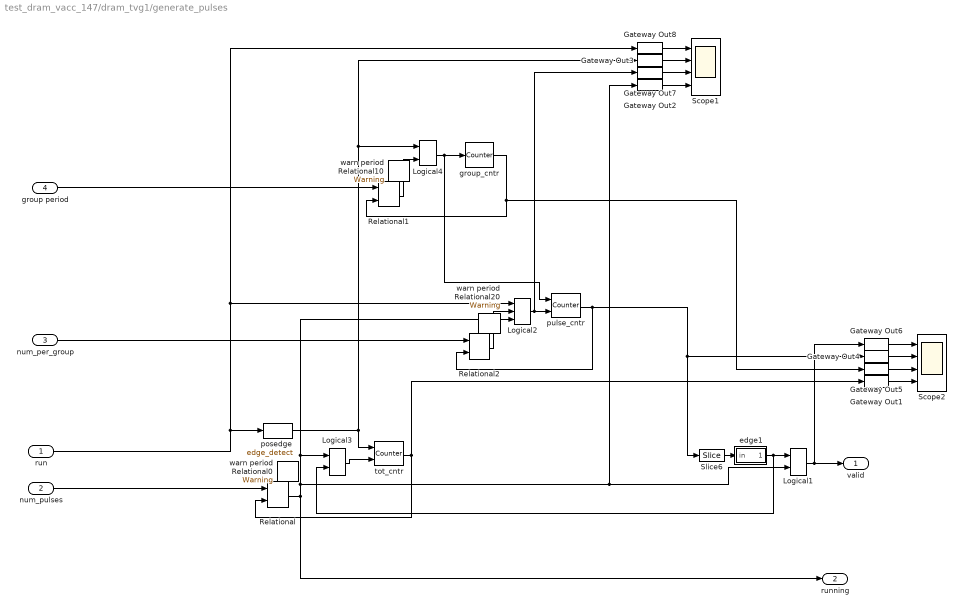
== system test_dram_vacc_147/dram_tvg1/generate_pulses ==
  run : Inport
  num_pulses : Inport  Port=2
  num_per_group : Inport  Port=3
  group period : Inport  Port=4
  Gateway Out{1..8} (8 alike) : xbsIndex_r4/Gateway Out  inherit_from_input=off  hdl_port=off  timing_constraint=None  locs_specified=off  LOCs={}  UseAsDAC=off  DACChannel='1'  block_type=gatewayout
      settings: xl_area=[0, 0, 0, 0, 0, 0, 0]
  Logical1 : xbsIndex_r4/Logical  logical_function=AND  inputs=2  en=off  latency=0  precision=Full  arith_type=Unsigned  n_bits=8  bin_pt=2  align_bp=on  dbl_ovrd=off  block_type=logical
      settings: xl_area=[0, 0, 0, 0, 0, 0, 0]
  Logical2 : xbsIndex_r4/Logical  logical_function=AND  inputs=3  en=off  latency=0  precision=Full  arith_type=Unsigned  n_bits=8  bin_pt=2  align_bp=on  dbl_ovrd=off  block_type=logical
      settings: xl_area=[0, 0, 0, 0, 0, 0, 0]
  Logical3 : xbsIndex_r4/Logical  logical_function=AND  inputs=2  en=off  latency=0  precision=Full  arith_type=Unsigned  n_bits=8  bin_pt=2  align_bp=on  dbl_ovrd=off  block_type=logical
      settings: xl_area=[0, 0, 0, 0, 0, 0, 0]
  Logical4 : xbsIndex_r4/Logical  logical_function=OR  inputs=2  en=off  latency=0  precision=Full  arith_type=Unsigned  n_bits=8  bin_pt=2  align_bp=off  dbl_ovrd=off  block_type=logical
      settings: xl_area=[0, 0, 0, 0, 0, 0, 0]
  Relational : xbsIndex_r4/Relational  mode=a>=b  en=off  latency=0  dbl_ovrd=off  block_type=relational
      settings: xl_area=[0, 0, 0, 0, 0, 0, 0]
  Relational1 : xbsIndex_r4/Relational  mode=a=b  en=off  latency=0  dbl_ovrd=off  block_type=relational
      settings: xl_area=[0, 0, 0, 0, 0, 0, 0]
  Relational2 : xbsIndex_r4/Relational  mode=a>b  en=off  latency=0  dbl_ovrd=off  block_type=relational
      settings: xl_area=[0, 0, 0, 0, 0, 0, 0]
  Scope1 : Scope  NumInputPorts=4
      settings: YMin=0~-1~0~0  YMax=1~1~1~1
  Scope2 : Scope  NumInputPorts=4
      settings: YMin=0.95~0~-1~-5  YMax=1.05~1~1~5
  Slice6 : xbsIndex_r4/Slice  nbits=1  boolean_output=on  mode=Lower Bit Location + Width  bit1=3  base1=LSB of Input  bit0=0  base0=LSB of Input  dbl_ovrd=off  block_type=slice
  edge1 : Subsystem  AncestorBlock=casper_library_misc/edge_detect  mask(edge_detect){edge=Both, polarity=Active High, x_in=[0 0.08 0.08 0.16 0.16 0.24 0.24 0.32 0.32 0.4], y_in=[-1 -1  1  1  1  1  1  1  1  1], x_out=[0.6 0.68 0.68 0.76 0.76 0.84 0.84 0.92 0.92 1], y_out=[-1 -1  1  1 -1 -1 -1 -1 -1 -1]}
      mask prompts: edge "Edge Type"; polarity "Output Polarity"; x_in "Input X Positions"; y_in "Input Y Positions"; x_out "Output X Positions"; y_out "Output Y Positions"
      mask help: Output is active for one-cycle after each edge of the specified type (i.e. rising, falling or both).
      mask init:
      | edge_detect_init(gcb,...
      |     'edge',edge,...
      |     'polarity',polarity,...
      |     'x_in',x_in,...
      |     'x_out',x_out,...
      |     'y_in',y_in,...
      |     'y_out',y_out);
      | 
      | x_in_num=str2num(getfield(getfield(get_param(gcb,'UserData'),'parameters'),'x_in'));
      | x_out_num=str2num(getfield(getfield(get_param(gcb,'UserData'),'parameters'),'x_out'));
      | y_in_num=str2num(getfield(getfield(get_param(gcb,'UserData'),'parameters'),'y_in'));
      | y_out_num=str2num(getfield(getfield(get_param(gcb,'UserData'),'parameters'),'y_out'));
      settings: AttributesFormatString=|
      | both edges
      | active high
      mask Help: Output is active for one-cycle after each edge of the specified type (i.e. rising, falling, or both).  Latency is zero.
      mask TypeOptions edge: Rising | Falling | Both
      mask TypeOptions polarity: Active High | Active Low
      mask Display:
      | plot(x_in_num,0.5+y_in_num*0.2);
      | plot(x_out_num,0.5+y_out_num*0.2);
  group_cntr : xbsIndex_r4/Counter  cnt_type=Free Running  cnt_to=1  operation=Up  start_count=1  cnt_by_val=1  arith_type=Unsigned  n_bits=32  bin_pt=0  load_pin=off  rst=on  en=off  explicit_period=on  period=1  dbl_ovrd=off  use_behavioral_HDL=off  implementation=Fabric  use_rpm=on  block_type=counter
      settings: xl_area=[0, 0, 0, 0, 0, 0, 0]
  posedge : casper_library_misc/edge_detect  edge=Rising  polarity=Active High  x_in=[0 0.08 0.08 0.16 0.16 0.24 0.24 0.32 0.32 0.4]  y_in="[-1 -1  1  1  1  1  1  1  1  1]"  x_out=[0.6 0.68 0.68 0.76 0.76 0.84 0.84 0.92 0.92 1]  y_out="[-1 -1  1  1 -1 -1 -1 -1 -1 -1]"
  pulse_cntr : xbsIndex_r4/Counter  cnt_type=Free Running  cnt_to=1  operation=Up  start_count=0  cnt_by_val=1  arith_type=Unsigned  n_bits=32  bin_pt=0  load_pin=off  rst=on  en=on  explicit_period=on  period=1  dbl_ovrd=off  use_behavioral_HDL=off  implementation=Fabric  use_rpm=on  block_type=counter
      settings: xl_area=[0, 0, 0, 0, 0, 0, 0]
  tot_cntr : xbsIndex_r4/Counter  cnt_type=Free Running  cnt_to=1  operation=Up  start_count=1  cnt_by_val=1  arith_type=Unsigned  n_bits=32  bin_pt=0  load_pin=off  rst=on  en=on  explicit_period=on  period=1  dbl_ovrd=off  use_behavioral_HDL=off  implementation=Fabric  use_rpm=on  block_type=counter
      settings: xl_area=[0, 0, 0, 0, 0, 0, 0]
  warn period Relational0 : xbsReplacements_r4/Warning  period=1
  warn period Relational10 : xbsReplacements_r4/Warning  period=1
  warn period Relational20 : xbsReplacements_r4/Warning  period=1
  valid : Outport
  running : Outport  Port=2
  wires:
  tot_cntr/1 -> Relational/2, Gateway Out1/1
  Slice6/1 -> edge1/1(in)
  run/1 -> posedge/1, Logical2/1, Gateway Out8/1
  Relational/1 -> Logical2/3, Logical3/1, Logical1/2, Gateway Out2/1, running/1
  num_pulses/1 -> Relational/1
  posedge/1 -> tot_cntr/1, Logical4/1, Gateway Out3/1
  group_cntr/1 -> Relational1/2, Gateway Out5/1
  Relational1/1 -> Logical4/2
  pulse_cntr/1 -> Relational2/2, Slice6/1, Gateway Out4/1
  Relational2/1 -> Logical2/2
  num_per_group/1 -> Relational2/1
  Logical2/1 -> pulse_cntr/2, Gateway Out7/1
  Logical4/1 -> group_cntr/1, pulse_cntr/1
  group period/1 -> Relational1/1
  Gateway Out5/1 -> Scope2/3
  Gateway Out4/1 -> Scope2/2
  Gateway Out6/1 -> Scope2/1
  Gateway Out1/1 -> Scope2/4
  Gateway Out7/1 -> Scope1/3
  Gateway Out3/1 -> Scope1/2
  Gateway Out8/1 -> Scope1/1
  Gateway Out2/1 -> Scope1/4
  edge1/1(out) -> Logical1/1, Logical3/2
  Logical1/1 -> valid/1, Gateway Out6/1
  Logical3/1 -> tot_cntr/2

== system test_dram_vacc_147/dram_tvg1/group_period ==
  sim_1 : Inport
  io_delay : xbsIndex_r4/Delay  rst=off  infoeditControl=Selection of Reset will increase slice count due to use of real FFs and instead of SRLs  en=off  latency=0  dbl_ovrd=off  reg_retiming=on  block_type=delay
  reint1 : xbsIndex_r4/Reinterpret  force_arith_type=on  arith_type=Unsigned  force_bin_pt=on  bin_pt=0  block_type=reinterpret
  slice_reg : xbsIndex_r4/Slice  nbits=32  boolean_output=off  mode=Lower Bit Location + Width  bit1=0  base1=MSB of Input  bit0=0  base0=LSB of Input  dbl_ovrd=off  block_type=slice
  test_dram_vacc_147_dram_tvg1_group_period_user_data_out : xbsIndex_r4/Gateway In  gui_display_data_type=Fixed-point  arith_type=Unsigned  n_bits=32  bin_pt=0  preci_type=Single  exp_width=8  frac_width=24  quantization="Round  (unbiased: +/- Inf)"  overflow=Saturate  period=1  dbl_ovrd=off  timing_constraint=None  locs_specified=off  LOCs={}  UseAsADC=off  ADCChannel='1'  inherit_from_input=off  hdl_port=on  block_type=gatewayin
  in_reg : Outport
  wires:
  test_dram_vacc_147_dram_tvg1_group_period_user_data_out/1 -> io_delay/1
  sim_1/1 -> test_dram_vacc_147_dram_tvg1_group_period_user_data_out/1
  io_delay/1 -> slice_reg/1
  slice_reg/1 -> reint1/1
  reint1/1 -> in_reg/1
